simulink model "Lab3ASimulinkClosedLoopDisturbance"  (R2018a)
settings: Solver=VariableStepAuto  StartTime=0.0  StopTime=600  RelTol=1e-6
settings Model: Creator=melab2  LastModifiedBy=melab2

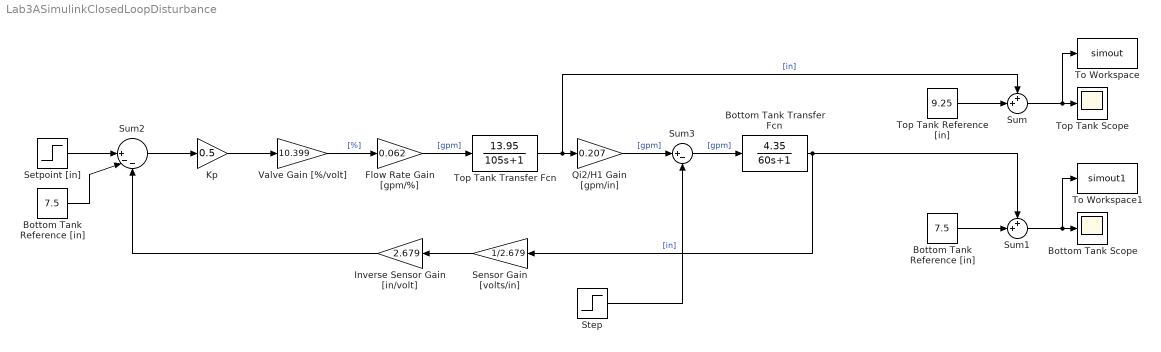
== system Lab3ASimulinkClosedLoopDisturbance ==
  Bottom Tank Transfer Fcn : TransferFcn  Numerator=[4.35]  Denominator=[60 1]
  Bottom Tank Reference [in] : Constant  Value=7.5
  "Bottom Tank Reference [in] " : Constant  Value=7.5
  Bottom Tank Scope : Scope
  Flow Rate Gain [gpm/%] : Gain  Gain=0.062
  Inverse Sensor Gain [in/volt] : Gain  Gain=2.679
  Kp : Gain  Gain=0.5
  Qi2/H1 Gain [gpm/in] : Gain  Gain=0.207
  Sensor Gain [volts/in] : Gain  Gain=1/2.679
  Setpoint [in] : Step  Time=0  After=7.5  SampleTime=0
  Step : Step  Time=10  SampleTime=0
  Sum : Sum  Inputs=++|
  Sum1 : Sum  Inputs=++|
  Sum2 : Sum  Inputs=||+--
  Sum3 : Sum  Inputs=|+-
  To Workspace : ToWorkspace  VariableName=simout  SampleTime=-1
  To Workspace1 : ToWorkspace  VariableName=simout1  SampleTime=-1
  Top Tank Transfer Fcn : TransferFcn  Numerator=[13.95]  Denominator=[105 1]
  "Top Tank Reference [in] " : Constant  Value=9.25
  Top Tank Scope : Scope
  Valve Gain [%/volt] : Gain  Gain=10.399
  wires:
  Top Tank Transfer Fcn/1 -> Sum/1, Qi2/H1 Gain [gpm/in]/1  "[in]"
  Flow Rate Gain [gpm/%]/1 -> Top Tank Transfer Fcn/1  "[gpm]"
  Valve Gain [%/volt]/1 -> Flow Rate Gain [gpm/%]/1  "[%]"
  "Bottom Tank Reference [in] "/1 -> Sum1/2
  Sum/1 -> To Workspace/1, Top Tank Scope/1
  Sum1/1 -> To Workspace1/1, Bottom Tank Scope/1
  "Top Tank Reference [in] "/1 -> Sum/2
  Bottom Tank Transfer Fcn/1 -> Sensor Gain [volts/in]/1, Sum1/1  "[in]"
  Setpoint [in]/1 -> Sum2/1
  Bottom Tank Reference [in]/1 -> Sum2/2
  Kp/1 -> Valve Gain [%/volt]/1
  Sum2/1 -> Kp/1
  Sum3/1 -> Bottom Tank Transfer Fcn/1  "[gpm]"
  Qi2/H1 Gain [gpm/in]/1 -> Sum3/1  "[gpm]"
  Sensor Gain [volts/in]/1 -> Inverse Sensor Gain [in/volt]/1
  Inverse Sensor Gain [in/volt]/1 -> Sum2/3
  Step/1 -> Sum3/2
